simulink model "Automated_features"  (R2021a)
settings: Solver=VariableStepAuto  StartTime=0.0  StopTime=10.0  RelTol=1e-3
undefined symbols (not defined in the file): sigbuilder_block
libraries: simulink x123
(part 1 of 2)
settings Model: Creator=99003762  LastModifiedBy=Dell
settings SolverCC: AlgebraicLoopSolver=TrustRegion
settings DebuggingCC: SFMachineParentedDataDiag=warning

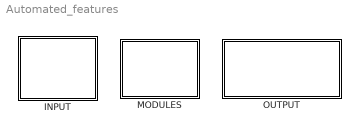
== system Automated_features ==
  INPUT : Subsystem
  MODULES : Subsystem
  OUTPUT : Subsystem

== system Automated_features/INPUT ==
  AIRBAG_INPUTS : Subsystem
  ALARM_INPUTS : Subsystem
  SEAT_RESTRAINT_INPUTS : Subsystem
  Wiper_INPUTS : Subsystem

== system Automated_features/MODULES ==
  AIRBAGSYSTEM : Subsystem
  ALARM_SYSTEM : Subsystem
  SeatBelt_MODULE : Subsystem
  WIPER_CONTROL : Subsystem
  tag scope: CushionAngle=global, FrontAngle=global, RearAngle=global, SeatAdj=global
  wires:
  SeatBelt_MODULE/4(CushionAdjustAngle) -> [CushionAngle]
  SeatBelt_MODULE/2(RearAdjustAngle) -> [RearAngle]
  SeatBelt_MODULE/3(SeatAdjust) -> [SeatAdj]
  SeatBelt_MODULE/1(FrontAdjustAngle) -> [FrontAngle]

== system Automated_features/OUTPUT ==
  AIRBAG_OUTPUTS : Subsystem
  ALARM_OUTPUT1 : Subsystem
  OUTPUT2 : Subsystem
  SeatBelt_OUTPUTS : Subsystem

== system Automated_features/INPUT/AIRBAG_INPUTS ==
  Signal Builder : Subsystem  Tag=STV Subsys  LoadFcn=sigbuilder_block('load');  StartFcn=sigbuilder_block('start');  StopFcn=sigbuilder_block('stop');  ClipboardFcn=sigbuilder_block('clipboard');  mask(Sigbuilder block){tuvar=[0:10]}
      mask help: Simulink:masks:SigbuilderBlock_MD
      mask init:
      | if ~strcmp(get_param(bdroot(gcbh),'SimulationStatus'),'stopped') tuvar = sigbuilder_block('maskInit'); end
      settings: CopyFcn=sigbuilder_block('copy');  DeleteFcn=sigbuilder_block('delete');  ModelCloseFcn=sigbuilder_block('modelClose');  PreSaveFcn=sigbuilder_block('preSave');  PauseFcn=sigbuilder_block('pause');  ContinueFcn=sigbuilder_block('continue');  NameChangeFcn=sigbuilder_block('namechange');  OpenFcn=sigbuilder_block('open',[437.6 199.2 550.4 400 ]);  CloseFcn=sigbuilder_block('close');
      mask Display: plot(0, 0, 100, 100,[2, 2, 32, 32, 2], [68, 8, 8, 68, 68],[32, 2], [38, 38], [32, 19, 2],[53, 60, 44], [32, 17, 17, 2],[16, 16, 31, 31]);txt = getActiveGroup(gcbh);text(2, 100, txt,'verticalAlignment', 'top');
  tag scope: Air_ACC=global, Driver_L=global, L_Front_1=global, L_Rear_1=global, R_Rear_=global, VehicleSpeed=global, YawRate=global
  wires:
  Signal Builder/1(Driver_L) -> [Driver_L]
  Signal Builder/2(L_Front_1) -> [L_Front_1]
  Signal Builder/3(L_Rear_1) -> [L_Rear_1]
  Signal Builder/4(R_Rear_) -> [R_Rear_]
  Signal Builder/5(VehicleSpeed) -> [VehicleSpeed]
  Signal Builder/6(Air_ACC) -> [Air_ACC]
  Signal Builder/7(YawRate) -> [YawRate]

== system Automated_features/INPUT/ALARM_INPUTS ==
  Signal Builder : Subsystem  Tag=STV Subsys  LoadFcn=sigbuilder_block('load');  StartFcn=sigbuilder_block('start');  StopFcn=sigbuilder_block('stop');  ClipboardFcn=sigbuilder_block('clipboard');  mask(Sigbuilder block){tuvar=[0:10]}
      mask help: Simulink:masks:SigbuilderBlock_MD
      mask init:
      | if ~strcmp(get_param(bdroot(gcbh),'SimulationStatus'),'stopped') tuvar = sigbuilder_block('maskInit'); end
      settings: CopyFcn=sigbuilder_block('copy');  DeleteFcn=sigbuilder_block('delete');  ModelCloseFcn=sigbuilder_block('modelClose');  PreSaveFcn=sigbuilder_block('preSave');  PauseFcn=sigbuilder_block('pause');  ContinueFcn=sigbuilder_block('continue');  NameChangeFcn=sigbuilder_block('namechange');  OpenFcn=sigbuilder_block('open',[403.5 199.2 550.5 359.55 ]);  CloseFcn=sigbuilder_block('close');
      mask Display: plot(0, 0, 100, 100,[2, 2, 32, 32, 2], [68, 8, 8, 68, 68],[32, 2], [38, 38], [32, 19, 2],[53, 60, 44], [32, 17, 17, 2],[16, 16, 31, 31]);txt = getActiveGroup(gcbh);text(2, 100, txt,'verticalAlignment', 'top');
  tag scope: AS_Doors=global, CAR_ON=global, Ignition=global, RKE=global
  wires:
  Signal Builder/1(AS_Doors) -> [AS_Doors]
  Signal Builder/2(Ignition) -> [Ignition]
  Signal Builder/3(Car_ON) -> [CAR_ON]
  Signal Builder/4(RKE) -> [RKE]

== system Automated_features/INPUT/SEAT_RESTRAINT_INPUTS ==
  tag scope: AdjustCushionAngle=global, AdjustFrontSeatAngle=global, AdjustRearSeatAngle=global, AdjustSeat=global, FrontSeat=global, HandleOn=global, ModeSelection=global, PowerSeat=global

== system Automated_features/INPUT/Wiper_INPUTS ==
  Signal Builder : Subsystem  Tag=STV Subsys  LoadFcn=sigbuilder_block('load');  StartFcn=sigbuilder_block('start');  StopFcn=sigbuilder_block('stop');  ClipboardFcn=sigbuilder_block('clipboard');  mask(Sigbuilder block){tuvar=[0:10]}
      mask help: Simulink:masks:SigbuilderBlock_MD
      mask init:
      | if ~strcmp(get_param(bdroot(gcbh),'SimulationStatus'),'stopped') tuvar = sigbuilder_block('maskInit'); end
      settings: CopyFcn=sigbuilder_block('copy');  DeleteFcn=sigbuilder_block('delete');  ModelCloseFcn=sigbuilder_block('modelClose');  PreSaveFcn=sigbuilder_block('preSave');  PauseFcn=sigbuilder_block('pause');  ContinueFcn=sigbuilder_block('continue');  NameChangeFcn=sigbuilder_block('namechange');  OpenFcn=sigbuilder_block('open',[437.6 199.2 550.4 400 ]);  CloseFcn=sigbuilder_block('close');
      mask Display: plot(0, 0, 100, 100,[2, 2, 32, 32, 2], [68, 8, 8, 68, 68],[32, 2], [38, 38], [32, 19, 2],[53, 60, 44], [32, 17, 17, 2],[16, 16, 31, 31]);txt = getActiveGroup(gcbh);text(2, 100, txt,'verticalAlignment', 'top');
  tag scope: FC_ManualInput=global, FW_Modes=global, WC_BackS=global, WC_FrontS=global, WC_Status=global
  wires:
  Signal Builder/1(FC_Modes) -> [FW_Modes]
  Signal Builder/2(FC_ManualInput) -> [FC_ManualInput]
  Signal Builder/3(WC_BackS) -> [WC_BackS]
  Signal Builder/4(WC_Fronts) -> [WC_FrontS]
  Signal Builder/5(WC_Status) -> [WC_Status]

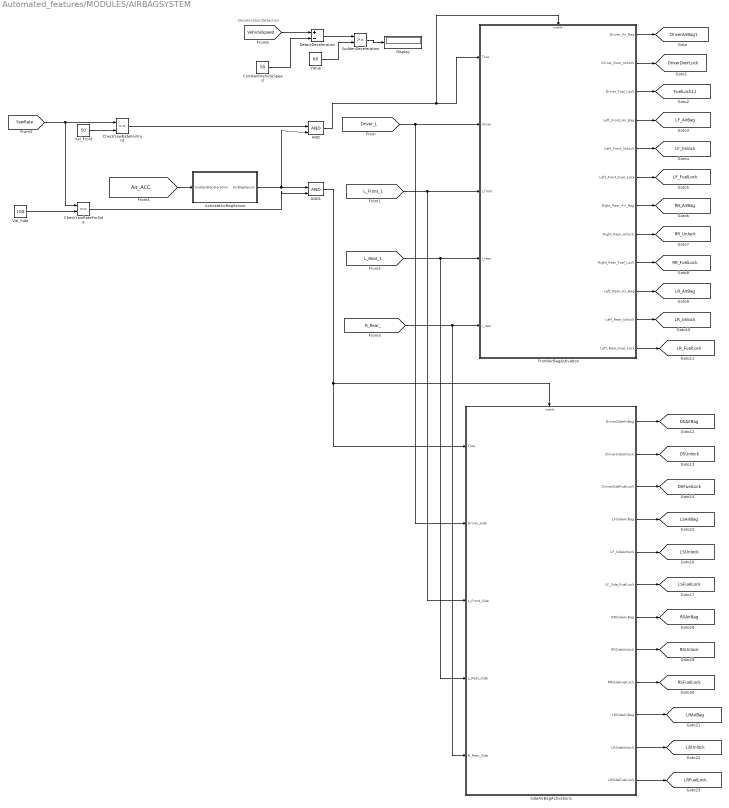
== system Automated_features/MODULES/AIRBAGSYSTEM ==
  note: DecelerationDetection
  AND : Logic  IconShape=distinctive  AllPortsSameDT=off  OutDataTypeStr=boolean
  AND1 : Logic  IconShape=distinctive  AllPortsSameDT=off  OutDataTypeStr=boolean
  ActivateAirBagSensor : MATLAB Function  TreatAsAtomicUnit=on
  CheckYawRateForFront : RelationalOperator  Operator===  OutDataTypeStr=boolean  RndMeth=Simplest
  CheckYawRateForSide : RelationalOperator  Operator===  OutDataTypeStr=boolean  RndMeth=Simplest
  ConstantVehicleSpeed : Constant  Value=50
  DetectDeceleration : Sum  Inputs=+-
  Display : Display
  FrontAirBagActivation : Subsystem  TreatAsAtomicUnit=on
  SideAirBagActivation1 : Subsystem  TreatAsAtomicUnit=on
  SuddenDeceleration : RelationalOperator  OutDataTypeStr=boolean  RndMeth=Simplest
  Val_Front : Constant  Value=50
  Val_Side : Constant  Value=100
  Value : Constant  Value=60
  tag scope: DSAirBag=global, DSFuelLock=global, DSUnlock=global, DriverAirBag1=global, DriverDoorLock=global, FuelLock11=global, LF_AirBag=global, LF_FuelLock=global, LF_Unlock=global, LRAirBag=global, LRFuelLock=global, LRUnlock=global, LR_AirBag=global, LR_FuelLock=global, LR_Unlock=global, LSAirBag=global, LSFuelLock=global, LSUnlock=global, RR_AirBag=global, RR_FuelLock=global, RR_Unlock=global, RSAirBag=global, RSFuelLock=global, RSUnlock=global
  wires:
  CheckYawRateForFront/1 -> AND/1
  AND1/1 -> SideAirBagActivation1/1(True), SideAirBagActivation1/Enable
  ActivateAirBagSensor/1(AirBagSensor) -> AND1/1, AND/2
  [VehicleSpeed] -> DetectDeceleration/1
  ConstantVehicleSpeed/1 -> DetectDeceleration/2
  AND/1 -> FrontAirBagActivation/1(True), FrontAirBagActivation/Enable
  [Air_ACC] -> ActivateAirBagSensor/1(SuddenDeceleration)
  Value/1 -> SuddenDeceleration/2
  DetectDeceleration/1 -> SuddenDeceleration/1
  SuddenDeceleration/1 -> Display/1
  [YawRate] -> CheckYawRateForSide/1, CheckYawRateForFront/1
  Val_Side/1 -> CheckYawRateForSide/2
  [Driver_L] -> FrontAirBagActivation/2(driver), SideAirBagActivation1/2(Driver_Side)
  Val_Front/1 -> CheckYawRateForFront/2
  [R_Rear_] -> SideAirBagActivation1/5(R_Rear_Side), FrontAirBagActivation/5(r_rear)
  [L_Rear_1] -> SideAirBagActivation1/4(L_Rear_Side), FrontAirBagActivation/4(l_rear)
  [L_Front_1] -> FrontAirBagActivation/3(l_front), SideAirBagActivation1/3(L_Front_Side)
  CheckYawRateForSide/1 -> AND1/2
  FrontAirBagActivation/1(Driver_Air_Bag) -> [DriverAirBag1]
  FrontAirBagActivation/2(Driver_Door_Unlock) -> [DriverDoorLock]
  FrontAirBagActivation/3(Driver_Fuel_Lock) -> [FuelLock11]
  FrontAirBagActivation/4(Left_Front_Air_Bag) -> [LF_AirBag]
  FrontAirBagActivation/5(Left_Front_Unlock) -> [LF_Unlock]
  FrontAirBagActivation/6(Left_Front_Fuel_Lock) -> [LF_FuelLock]
  FrontAirBagActivation/7(Right_Rear_Air_Bag) -> [RR_AirBag]
  FrontAirBagActivation/8(Right_Rear_Unlock) -> [RR_Unlock]
  FrontAirBagActivation/9(Right_Rear_Fuel_Lock) -> [RR_FuelLock]
  FrontAirBagActivation/10(Left_Rear_Air_Bag) -> [LR_AirBag]
  FrontAirBagActivation/11(Left_Rear_Unlock) -> [LR_Unlock]
  FrontAirBagActivation/12(Left_Rear_Fuel_Lock) -> [LR_FuelLock]
  SideAirBagActivation1/1(DriverSideAirBag) -> [DSAirBag]
  SideAirBagActivation1/2(DriverSideUnlock) -> [DSUnlock]
  SideAirBagActivation1/3(DriverSideFuelLock) -> [DSFuelLock]
  SideAirBagActivation1/4(LFSideAirBag) -> [LSAirBag]
  SideAirBagActivation1/5(LF_SideUnlock) -> [LSUnlock]
  SideAirBagActivation1/6(LF_Side_FuelLock) -> [LSFuelLock]
  SideAirBagActivation1/7(RRSideAirBag) -> [RSAirBag]
  SideAirBagActivation1/8(RRSideUnlock) -> [RSUnlock]
  SideAirBagActivation1/9(RRSideFuelLock) -> [RSFuelLock]
  SideAirBagActivation1/10(LRSideAirBag) -> [LRAirBag]
  SideAirBagActivation1/11(LRSideUnlock) -> [LRUnlock]
  SideAirBagActivation1/12(LRSideFuelLock) -> [LRFuelLock]

== system Automated_features/MODULES/ALARM_SYSTEM ==
  AND : Logic  Inputs=3  IconShape=distinctive  AllPortsSameDT=off  OutDataTypeStr=boolean
  AND1 : Logic  Inputs=3  IconShape=distinctive  AllPortsSameDT=off  OutDataTypeStr=boolean
  AND2 : Logic  IconShape=distinctive  AllPortsSameDT=off  OutDataTypeStr=boolean
  AND3 : Logic  IconShape=distinctive  AllPortsSameDT=off  OutDataTypeStr=boolean
  ARMED : Stateflow chart  TreatAsAtomicUnit=on
  Compare To Constant : simulink/Logic and Bit Operations/Compare To Constant  relop===  const=0  OutDataTypeStr=boolean
  Compare To Constant2 : simulink/Logic and Bit Operations/Compare To Constant  relop===  const=1  OutDataTypeStr=boolean
  Compare To Constant3 : simulink/Logic and Bit Operations/Compare To Constant  relop===  const=1  OutDataTypeStr=boolean
  Compare To Zero : simulink/Logic and Bit Operations/Compare To Zero  relop===  OutDataTypeStr=boolean
  Compare To Zero1 : simulink/Logic and Bit Operations/Compare To Zero  relop===  OutDataTypeStr=boolean
  Constant : Constant
  Constant1 : Constant
  Constant2 : Constant
  Constant3 : Constant  Value=0
  Display : Display
  Main_Alarm : Subsystem  Commented=on
  NAND : Logic  Operator=NAND  IconShape=distinctive  AllPortsSameDT=off  OutDataTypeStr=boolean
  Pre_Alarm : Stateflow chart  TreatAsAtomicUnit=on
  Slider Switch : SliderSwitchBlock  Commented=on
      settings: Values={{'Off', 'On'}, [1 0]}
  Switch : Switch  Criteria=u2 ~= 0
  Switch1 : Switch  Criteria=u2 ~= 0
  Switch2 : Switch  Criteria=u2 ~= 0
  tag scope: Alarm_ARMED=global, Disarmed=global, Prealarm_ARMED=global
  wires:
  [RKE] -> AND1/2, Compare To Zero/1, AND2/2  "RKE"
  Constant/1 -> Switch/1
  Constant1/1 -> Switch1/1
  Compare To Zero1/1 -> AND3/2
  Compare To Constant3/1 -> NAND/1
  [CAR_ON] -> AND/2
  Compare To Zero/1 -> AND3/1
  AND2/1 -> ARMED/1(data)
  Pre_Alarm/1(data1) -> Switch1/2
  Compare To Constant/1 -> AND2/1
  AND1/1 -> Switch/2
  [Ignition] -> Compare To Constant2/1, AND/1
  AND/1 -> Compare To Constant/1
  Compare To Constant2/1 -> AND1/1
  Switch/1 -> Switch2/2, [Disarmed]
  Switch1/1 -> [Prealarm_ARMED]
  ARMED/1(data1) -> AND1/3, Compare To Constant3/1
  AND3/1 -> Pre_Alarm/1(data)
  [AS_Doors] -> Display/1, Compare To Zero1/1, AND/3
  Constant2/1 -> Switch2/1
  Switch2/1 -> NAND/2
  NAND/1 -> [Alarm_ARMED]
  Constant3/1 -> Switch2/3

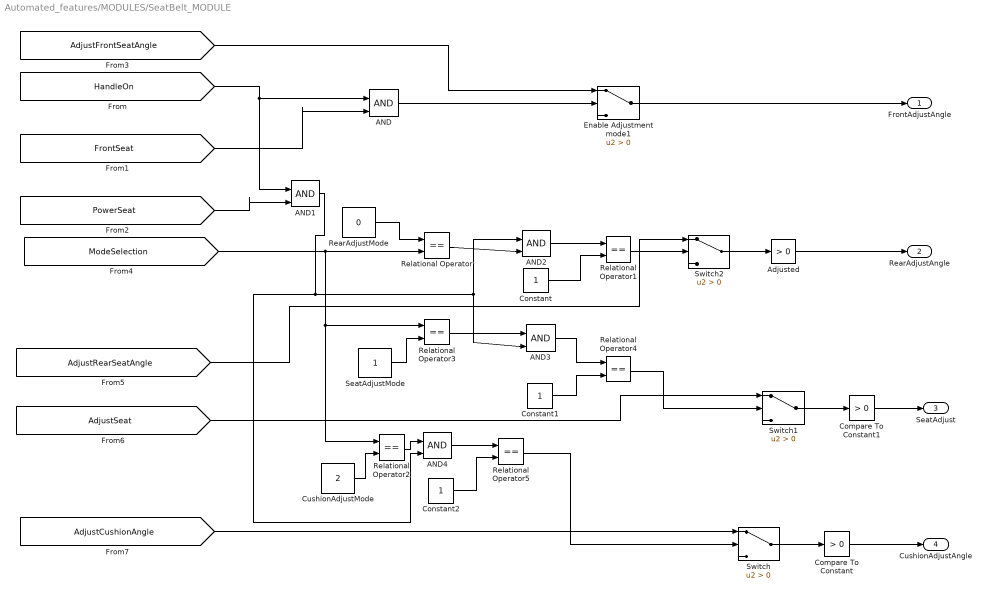
== system Automated_features/MODULES/SeatBelt_MODULE ==
  AND{,1..4} (5 alike) : Logic  IconShape=distinctive  AllPortsSameDT=off  OutDataTypeStr=boolean
  Adjusted : simulink/Logic and Bit Operations/Compare To Constant  relop=>  const=0  OutDataTypeStr=boolean
  Compare To Constant : simulink/Logic and Bit Operations/Compare To Constant  relop=>  const=0  OutDataTypeStr=boolean
  Compare To Constant1 : simulink/Logic and Bit Operations/Compare To Constant  relop=>  const=0  OutDataTypeStr=boolean
  Constant : Constant
  Constant1 : Constant
  Constant2 : Constant
  CushionAdjustMode : Constant  Value=2
  Enable Adjustment mode1 : Switch  Criteria=u2 > Threshold
  RearAdjustMode : Constant  Value=0
  Relational Operator{,1..5} (6 alike) : RelationalOperator  Operator===  OutDataTypeStr=boolean  RndMeth=Simplest
  SeatAdjustMode : Constant
  Switch : Switch  Criteria=u2 > Threshold
  Switch1 : Switch  Criteria=u2 > Threshold
  Switch2 : Switch  Criteria=u2 > Threshold
  FrontAdjustAngle : Outport
  RearAdjustAngle : Outport  Port=2
  SeatAdjust : Outport  Port=3
  CushionAdjustAngle : Outport  Port=4
  wires:
  AND3/1 -> Relational Operator4/1
  Compare To Constant/1 -> CushionAdjustAngle/1
  AND1/1 -> AND4/2, AND2/1, AND3/2
  [HandleOn] -> AND1/1, AND/1
  Switch2/1 -> Adjusted/1
  RearAdjustMode/1 -> Relational Operator/1
  [AdjustCushionAngle] -> Switch/1
  AND2/1 -> Relational Operator1/1
  AND/1 -> Enable Adjustment mode1/2
  Relational Operator2/1 -> AND4/1
  Compare To Constant1/1 -> SeatAdjust/1
  Constant/1 -> Relational Operator1/2
  [AdjustSeat] -> Switch1/1
  Relational Operator4/1 -> Switch1/2
  Switch/1 -> Compare To Constant/1
  Switch1/1 -> Compare To Constant1/1
  Relational Operator/1 -> AND2/2
  [FrontSeat] -> AND/2
  [AdjustRearSeatAngle] -> Switch2/1
  [ModeSelection] -> Relational Operator/2, Relational Operator2/1, Relational Operator3/1
  AND4/1 -> Relational Operator5/1
  Relational Operator3/1 -> AND3/1
  SeatAdjustMode/1 -> Relational Operator3/2
  Constant2/1 -> Relational Operator5/2
  Constant1/1 -> Relational Operator4/2
  [AdjustFrontSeatAngle] -> Enable Adjustment mode1/1
  Relational Operator1/1 -> Switch2/2
  Relational Operator5/1 -> Switch/2
  CushionAdjustMode/1 -> Relational Operator2/2
  [PowerSeat] -> AND1/2
  Adjusted/1 -> RearAdjustAngle/1
  Enable Adjustment mode1/1 -> FrontAdjustAngle/1

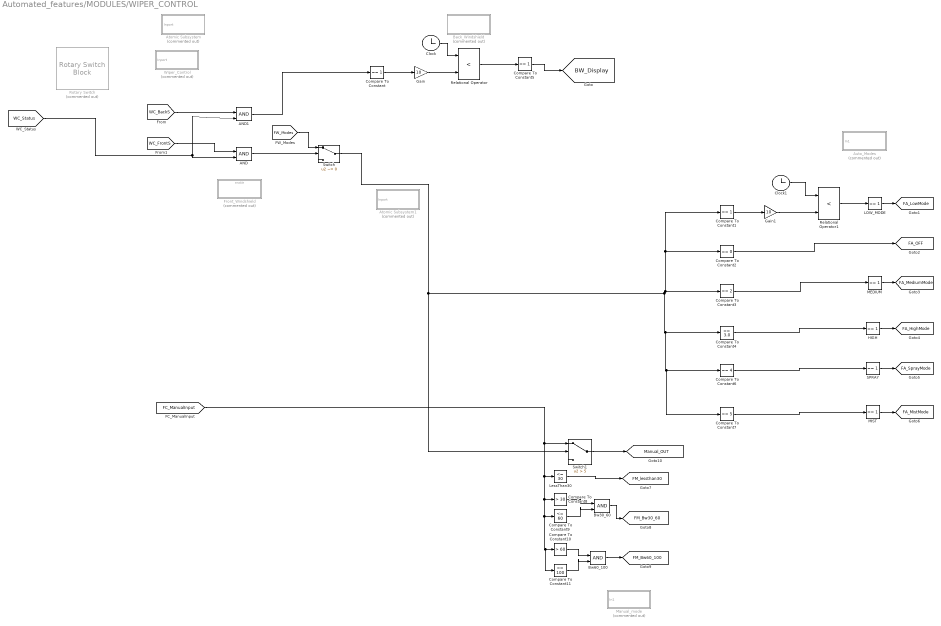
== system Automated_features/MODULES/WIPER_CONTROL ==
  AND : Logic  IconShape=distinctive  AllPortsSameDT=off  OutDataTypeStr=boolean
  AND1 : Logic  IconShape=distinctive  AllPortsSameDT=off  OutDataTypeStr=boolean
  Atomic Subsystem : Subsystem  Commented=on  TreatAsAtomicUnit=on
  Atomic Subsystem1 : Subsystem  Commented=on  TreatAsAtomicUnit=on
  Auto_Modes : Subsystem  Commented=on
  Back_Windshield : Subsystem  Commented=on  TreatAsAtomicUnit=on
  Bw30_60 : Logic  IconShape=distinctive  AllPortsSameDT=off  OutDataTypeStr=boolean
  Bw60_100 : Logic  IconShape=distinctive  AllPortsSameDT=off  OutDataTypeStr=boolean
  Clock : Clock
      settings: Decimation=5
  Clock1 : Clock
      settings: Decimation=5
  Compare To Constant : simulink/Logic and Bit Operations/Compare To Constant  relop===  const=1  OutDataTypeStr=boolean
  Compare To Constant1 : simulink/Logic and Bit Operations/Compare To Constant  relop===  const=1  OutDataTypeStr=boolean
  Compare To Constant10 : simulink/Logic and Bit Operations/Compare To Constant  relop=>  const=60  OutDataTypeStr=boolean
  Compare To Constant11 : simulink/Logic and Bit Operations/Compare To Constant  relop=<=  const=100  OutDataTypeStr=boolean
  Compare To Constant2 : simulink/Logic and Bit Operations/Compare To Constant  relop===  const=0  OutDataTypeStr=boolean
  Compare To Constant3 : simulink/Logic and Bit Operations/Compare To Constant  relop===  const=2  OutDataTypeStr=boolean
  Compare To Constant4 : simulink/Logic and Bit Operations/Compare To Constant  relop===  const=3.0  OutDataTypeStr=boolean
  Compare To Constant5 : simulink/Logic and Bit Operations/Compare To Constant  relop===  const=1  OutDataTypeStr=boolean
  Compare To Constant6 : simulink/Logic and Bit Operations/Compare To Constant  relop===  const=4  OutDataTypeStr=boolean
  Compare To Constant7 : simulink/Logic and Bit Operations/Compare To Constant  relop===  const=5  OutDataTypeStr=boolean
  Compare To Constant8 : simulink/Logic and Bit Operations/Compare To Constant  relop=>  const=30  OutDataTypeStr=boolean
  Compare To Constant9 : simulink/Logic and Bit Operations/Compare To Constant  relop=<=  const=60  OutDataTypeStr=boolean
  Front_Windshield : Subsystem  Commented=on  TreatAsAtomicUnit=on
  Gain : Gain  Gain=10
  Gain1 : Gain  Gain=10
  HIGH : simulink/Logic and Bit Operations/Compare To Constant  relop===  const=1  OutDataTypeStr=boolean
  LOW_MODE : simulink/Logic and Bit Operations/Compare To Constant  relop===  const=1  OutDataTypeStr=boolean
  LessThan30 : simulink/Logic and Bit Operations/Compare To Constant  relop=<=  const=30  OutDataTypeStr=boolean
  MEDIUM : simulink/Logic and Bit Operations/Compare To Constant  relop===  const=1  OutDataTypeStr=boolean
  MIST : simulink/Logic and Bit Operations/Compare To Constant  relop===  const=1  OutDataTypeStr=boolean
  Manual_mode : Subsystem  Commented=on
  Relational Operator : RelationalOperator  Operator=<  OutDataTypeStr=boolean  RndMeth=Simplest
  Relational Operator1 : RelationalOperator  Operator=<  OutDataTypeStr=boolean  RndMeth=Simplest
  Rotary Switch : RotarySwitchBlock  Commented=on
      settings: Values={{'Off', 'Accessory', 'Ignition'}, [0 1 2]}
  SPRAY : simulink/Logic and Bit Operations/Compare To Constant  relop===  const=1  OutDataTypeStr=boolean
  Switch : Switch  Criteria=u2 ~= 0
  Switch1 : Switch  Criteria=u2 > Threshold  Threshold=5
  Wiper_Control : Subsystem  Commented=on  TreatAsAtomicUnit=on
  tag scope: BW_Display=global, FA_HighMode=global, FA_LowMode=global, FA_MediumMode=global, FA_MistMode=global, FA_OFF=global, FA_SprayMode=global, FM_Bw30_60=global, FM_Bw60_100=global, FM_lessthan30=global, Manual_OUT=global
  wires:
  [WC_Status] -> AND1/2, AND/2
  [WC_BackS] -> AND1/1
  [WC_FrontS] -> AND/1
  Compare To Constant/1 -> Gain/1
  Relational Operator/1 -> Compare To Constant5/1
  Compare To Constant5/1 -> [BW_Display]
  Gain/1 -> Relational Operator/2
  Clock/1 -> Relational Operator/1
  AND1/1 -> Compare To Constant/1
  AND/1 -> Switch/2
  [FW_Modes] -> Switch/1
  Compare To Constant6/1 -> SPRAY/1
  MEDIUM/1 -> [FA_MediumMode]
  HIGH/1 -> [FA_HighMode]
  LOW_MODE/1 -> [FA_LowMode]
  Relational Operator1/1 -> LOW_MODE/1
  Clock1/1 -> Relational Operator1/1
  Gain1/1 -> Relational Operator1/2
  SPRAY/1 -> [FA_SprayMode]
  MIST/1 -> [FA_MistMode]
  Compare To Constant7/1 -> MIST/1
  Compare To Constant2/1 -> [FA_OFF]
  Compare To Constant1/1 -> Gain1/1
  Switch1/1 -> [Manual_OUT]
  [FC_ManualInput] -> Compare To Constant11/1, Compare To Constant10/1, Compare To Constant9/1, Compare To Constant8/1, LessThan30/1, Switch1/1
  Compare To Constant9/1 -> Bw30_60/2
  Switch/1 -> Switch1/2, Compare To Constant7/1, Compare To Constant6/1, Compare To Constant4/1, Compare To Constant3/1, Compare To Constant1/1, Compare To Constant2/1
  LessThan30/1 -> [FM_lessthan30]
  Compare To Constant10/1 -> Bw60_100/1
  Compare To Constant8/1 -> Bw30_60/1
  Compare To Constant11/1 -> Bw60_100/2
  Bw60_100/1 -> [FM_Bw60_100]
  Bw30_60/1 -> [FM_Bw30_60]
  Compare To Constant3/1 -> MEDIUM/1
  Compare To Constant4/1 -> HIGH/1

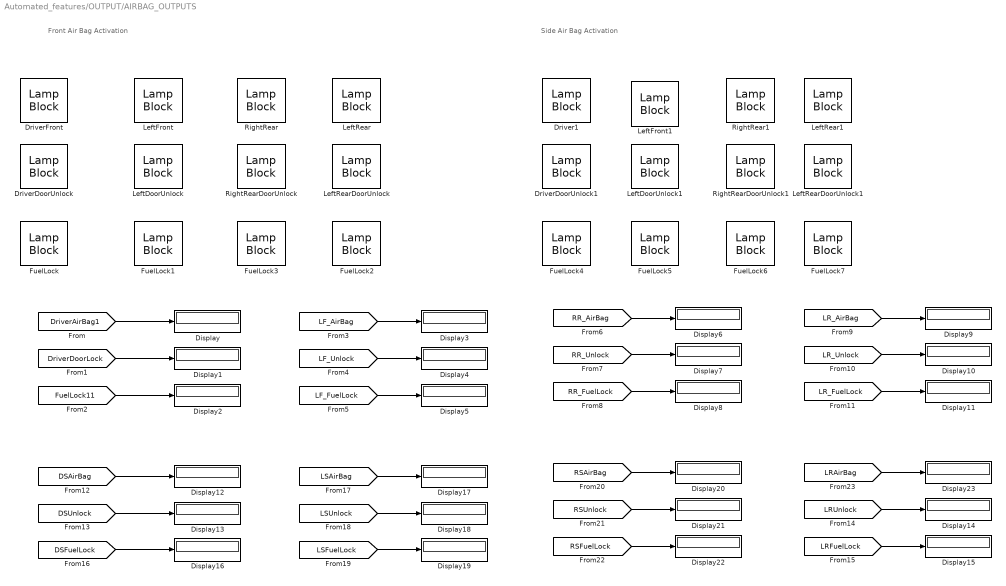
== system Automated_features/OUTPUT/AIRBAG_OUTPUTS ==
  note: Front Air Bag Activation
  note: Side Air Bag Activation
  Display{,1..23} (24 alike) : Display
  Driver1 : LampBlock
  DriverDoorUnlock : LampBlock
  DriverDoorUnlock1 : LampBlock
  DriverFront : LampBlock  Icon=Circle
  FuelLock{,1..7} (8 alike) : LampBlock
  LeftDoorUnlock : LampBlock
  LeftDoorUnlock1 : LampBlock
  LeftFront : LampBlock
  LeftFront1 : LampBlock
  LeftRear : LampBlock
  LeftRear1 : LampBlock
  LeftRearDoorUnlock : LampBlock
  LeftRearDoorUnlock1 : LampBlock
  RightRear : LampBlock
  RightRear1 : LampBlock
  RightRearDoorUnlock : LampBlock
  RightRearDoorUnlock1 : LampBlock
  wires:
  [DriverAirBag1] -> Display/1
  [DriverDoorLock] -> Display1/1
  [FuelLock11] -> Display2/1
  [LF_AirBag] -> Display3/1
  [LF_Unlock] -> Display4/1
  [LF_FuelLock] -> Display5/1
  [RR_AirBag] -> Display6/1
  [RR_Unlock] -> Display7/1
  [RR_FuelLock] -> Display8/1
  [LR_AirBag] -> Display9/1
  [LR_Unlock] -> Display10/1
  [LR_FuelLock] -> Display11/1
  [DSFuelLock] -> Display16/1
  [LRAirBag] -> Display23/1
  [RSUnlock] -> Display21/1
  [RSAirBag] -> Display20/1
  [RSFuelLock] -> Display22/1
  [DSUnlock] -> Display13/1
  [LSUnlock] -> Display18/1
  [LRUnlock] -> Display14/1
  [LSFuelLock] -> Display19/1
  [LSAirBag] -> Display17/1
  [LRFuelLock] -> Display15/1
  [DSAirBag] -> Display12/1

== system Automated_features/OUTPUT/ALARM_OUTPUT1 ==
  note: OUTPUTS
  Display : Display
  Display1 : Display
  Display2 : Display
  Lamp : LampBlock
  wires:
  [Disarmed] -> Display2/1
  [Prealarm_ARMED] -> Display1/1
  [Alarm_ARMED] -> Display/1

== system Automated_features/OUTPUT/OUTPUT2 ==
  note: BACK WINDSHIELD
  note: FRONT WINDSHIELD AUTOMODES
  note: FRONT WINDSHIELD MANUAL MANUAL OUTPUT
  Display{,1..10} (11 alike) : Display
  Lamp{,1..8} (9 alike) : LampBlock
  wires:
  [BW_Display] -> Display/1
  [FM_lessthan30] -> Display1/1
  [FM_Bw30_60] -> Display2/1
  [FM_Bw60_100] -> Display3/1
  [FA_LowMode] -> Display4/1
  [FA_MediumMode] -> Display5/1
  [FA_HighMode] -> Display6/1
  [FA_MistMode] -> Display7/1
  [FA_OFF] -> Display8/1
  [FA_SprayMode] -> Display9/1
  [Manual_OUT] -> Display10/1

== system Automated_features/OUTPUT/SeatBelt_OUTPUTS ==
  Display{,1..3} (4 alike) : Display
  wires:
  [RearAngle] -> Display1/1
  [SeatAdj] -> Display2/1
  [FrontAngle] -> Display/1
  [CushionAngle] -> Display3/1

== system Automated_features/INPUT/AIRBAG_INPUTS/Signal Builder ==
  Demux : Demux  Tag=STV Demux  Outputs=7
      settings: DisplayOption=none
  FromWs : FromWorkspace  Tag=STV FromWs  VariableName=tuvar
      SigBuilderData=|
      | common.afterFinalStr = 'Extrapolate'
      | common.sampleTime = 0
      | dataSet.timeRange = [0 10]
      | dataSet.name = 'Group 1'
      | sbobj.Groups.Name = 'Group 1'
      | sbobj.Groups.Signals(1).Name = 'Driver_L'
      | sbobj.Groups.Signals(1).XData = [0 1 2 3 4 5 6 7 10]
      | sbobj.Groups.Signals(1).YData = [0 1 1 1 1 1 1 0 0]
      | sbobj.Groups.Signals(2).Name = 'L_Front_1'
      | sbobj.Groups.Signals(2).XData = [0 1 2 3 4 5 6 7 10]
      | sbobj.Groups.Signals(2).YData = [0 0 0 0 0 0 0 0 0]
      | sbobj.Groups.Signals(3).Name = 'L_Rear_1'
      | sbobj.Groups.Signals(3).XData = [0 1 2 3 4 5 6 7 10]
      | sbobj.Groups.Signals(3).YData = [0 0 0 0 0 0 0 0 0]
      | sbobj.Groups.Signals(4).Name = 'R_Rear_'
      | sbobj.Groups.Signals(4).XData = [0 1 2 3 4 5 6 7 10]
      | sbobj.Groups.Signals(4).YData = [0 0 0 0 0 0 0 1 1]
      | sbobj.Groups.Signals(5).Name = 'VehicleSpeed'
      | sbobj.Groups.Signals(5).XData = [0 1 2 3 4 5 6 7 10]
      | sbobj.Groups.Signals(5).YData = [0 50 50 140 140 140 140 140 140]
      | sbobj.Groups.Signals(6).Name = 'Air_ACC'
      | sbobj.Groups.Signals(6).XData = [0 1 2 3 4 5 6 7 10]
      | sbobj.Groups.Signals(6).YData = [0 0 0 1 1 1 1 1 1]
      | sbobj.Groups.Signals(7).Name = 'YawRate'
      | sbobj.Groups.Signals(7).XData = [0 1 2 3 4 5 6 7 8 10]
      | sbobj.Groups.Signals(7).YData = [0 50 50 50 50 100 100 50 100 100]
  Driver_L : Outport  Tag=STV Outport
  L_Front_1 : Outport  Tag=STV Outport  Port=2
  L_Rear_1 : Outport  Tag=STV Outport  Port=3
  R_Rear_ : Outport  Tag=STV Outport  Port=4
  VehicleSpeed : Outport  Tag=STV Outport  Port=5
  Air_ACC : Outport  Tag=STV Outport  Port=6
  YawRate : Outport  Tag=STV Outport  Port=7
  wires:
  FromWs/1 -> Demux/1
  Demux/1 -> Driver_L/1
  Demux/2 -> L_Front_1/1
  Demux/3 -> L_Rear_1/1
  Demux/4 -> R_Rear_/1
  Demux/5 -> VehicleSpeed/1
  Demux/6 -> Air_ACC/1
  Demux/7 -> YawRate/1

== system Automated_features/INPUT/ALARM_INPUTS/Signal Builder ==
  Demux : Demux  Tag=STV Demux
      settings: DisplayOption=none
  FromWs : FromWorkspace  Tag=STV FromWs  VariableName=tuvar
      SigBuilderData=|
      | common.afterFinalStr = 'Extrapolate'
      | common.sampleTime = 0
      | dataSet.timeRange = [0 12]
      | dataSet.name = 'Group 1'
      | sbobj.Groups.Name = 'Group 1'
      | sbobj.Groups.Signals(1).Name = 'AS_Doors'
      | sbobj.Groups.Signals(1).XData = [0 1 2 3 4 5 6 7 8 9 10 11 12]
      | sbobj.Groups.Signals(1).YData = [0 1 1 1 1 1 1 1 1 1 1 1 1]
      | sbobj.Groups.Signals(2).Name = 'Ignition'
      | sbobj.Groups.Signals(2).XData = [0 1 2 3 4 5 6 7 8 9 10 11 12]
      | sbobj.Groups.Signals(2).YData = [0 1 1 1 1 1 1 1 1 1 1 1 1]
      | sbobj.Groups.Signals(3).Name = 'Car_ON'
      | sbobj.Groups.Signals(3).XData = [0 1 2 3 4 5 6 7 8 9 10 11 12]
      | sbobj.Groups.Signals(3).YData = [0 1 1 1 1 1 1 1 1 1 1 1 1]
      | sbobj.Groups.Signals(4).Name = 'RKE'
      | sbobj.Groups.Signals(4).XData = [0 1 2 3 4 5 6 7 8 9 10 11 12]
      | sbobj.Groups.Signals(4).YData = [0 1 1 1 1 1 2 2 2 2 2 2 2]
      | sbobj.Groups.TimeRange = [0 12]
  AS_Doors : Outport  Tag=STV Outport
  Ignition : Outport  Tag=STV Outport  Port=2
  Car_ON : Outport  Tag=STV Outport  Port=3
  RKE : Outport  Tag=STV Outport  Port=4
  wires:
  FromWs/1 -> Demux/1
  Demux/1 -> AS_Doors/1
  Demux/2 -> Ignition/1
  Demux/3 -> Car_ON/1
  Demux/4 -> RKE/1

== system Automated_features/INPUT/Wiper_INPUTS/Signal Builder ==
  Demux : Demux  Tag=STV Demux  Outputs=5
      settings: DisplayOption=none
  FromWs : FromWorkspace  Tag=STV FromWs  VariableName=tuvar
      SigBuilderData=|
      | common.afterFinalStr = 'Extrapolate'
      | common.sampleTime = 0
      | dataSet.timeRange = [0 10]
      | dataSet.name = 'Group 1'
      | sbobj.Groups.Name = 'Group 1'
      | sbobj.Groups.Signals(1).Name = 'FC_Modes'
      | sbobj.Groups.Signals(1).XData = [0 1 2 3 4 5 6 7 8 9 10 11 12 13 14 15 16 17 18 19 20 21 22 23 24 25 26 27 28 29 30 31 32 33 34 35 36 37 38 39 40 41 42 43]
      | sbobj.Groups.Signals(1).YData = [0 1 1 1 1 1 1 1 1 1 1 1 2 2 2 2 2 2 2 2 3 3 3 3 3 4 4 4 4 4 5 5 5 6 6 6 6 6 6 6 6 6 6 6]
      | sbobj.Groups.Signals(2).Name = 'FC_ManualInput'
      | sbobj.Groups.Signals(2).XData = [0 1 2 3 4 5 6 7 8 9 10 11 12 13 14 15 16 17 18 19 20 21 22 23 24 25 26 27 28 29 30 31 32 33 34 35 36 37 38 39 40 41 42 43]
      | sbobj.Groups.Signals(2).YData = [0 0 0 0 0 0 0 0 0 0 0 0 0 0 0 0 0 0 0 0 0 0 0 0 0 0 0 0 0 0 0 0 0 0 15 20 36 50 65 69 80 85 90 98]
      | sbobj.Groups.Signals(3).Name = 'WC_BackS'
      | sbobj.Groups.Signals(3).XData = [0 1 2 3 4 5 6 7 8 9 10 11 12 13 14 15 16 17 18 19 20 21 22 23 24 25 26 27 28 29 30 31 32 33 34 35 36 37 38 39 40 41 42 43]
      | sbobj.Groups.Signals(3).YData = [0 1 1 1 1 1 1 1 1 1 1 1 0 0 0 0 0 0 0 0 0 0 0 0 0 0 0 0 0 0 0 0 0 0 0 0 0 0 0 0 0 0 0 0]
      | sbobj.Groups.Signals(4).Name = 'WC_Fronts'
      | sbobj.Groups.Signals(4).XData = [0 1 2 3 4 5 6 7 8 9 10 11 12 13 14 15 16 17 18 19 20 21 22 23 24 25 26 27 28 29 30 31 32 33 34 35 36 37 38 39 40 41 42 43]
      | sbobj.Groups.Signals(4).YData = [0 1 1 1 1 1 1 1 1 1 1 1 1 1 1 1 1 1 1 1 1 1 1 1 1 1 1 1 1 1 1 1 1 1 1 1 1 1 1 1 1 1 1 1]
      | sbobj.Groups.Signals(5).Name = 'WC_Status'
      | sbobj.Groups.Signals(5).XData = [0 1 2 3 4 5 6 7 8 9 10 11 12 13 14 15 16 17 18 19 20 21 22 23 24 25 26 27 28 29 30 31 32 33 34 35 36 37 38 39 40 41 42 43]
      | sbobj.Groups.Signals(5).YData = [0 1 1 1 1 1 1 1 1 1 1 1 1 1 1 1 1 1 1 1 1 1 1 1 1 1 1 1 1 1 1 1 1 1 1 1 1 1 1 1 1 1 1 1]
  FC_Modes : Outport  Tag=STV Outport
  FC_ManualInput : Outport  Tag=STV Outport  Port=2
  WC_BackS : Outport  Tag=STV Outport  Port=3
  WC_Fronts : Outport  Tag=STV Outport  Port=4
  WC_Status : Outport  Tag=STV Outport  Port=5
  wires:
  FromWs/1 -> Demux/1
  Demux/1 -> FC_Modes/1
  Demux/2 -> FC_ManualInput/1
  Demux/3 -> WC_BackS/1
  Demux/4 -> WC_Fronts/1
  Demux/5 -> WC_Status/1

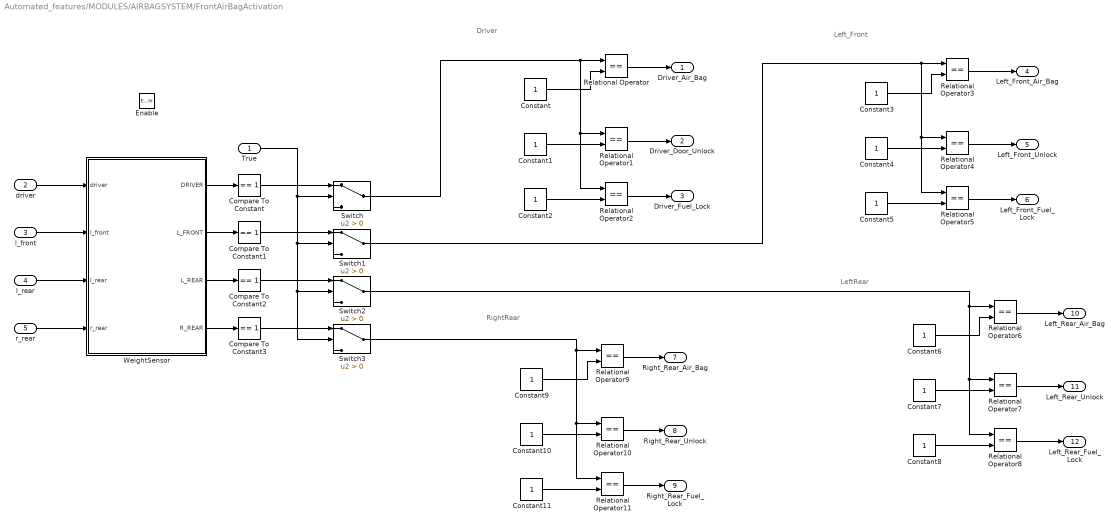
== system Automated_features/MODULES/AIRBAGSYSTEM/FrontAirBagActivation ==
  note: RightRear
  note: LeftRear
  note: Left_Front
  note: Driver
  True : Inport
  driver : Inport  Port=2
  l_front : Inport  Port=3
  l_rear : Inport  Port=4
  r_rear : Inport  Port=5
  Enable : EnablePort
  Compare To Constant{,1..3} (4 alike) : simulink/Logic and Bit Operations/Compare To Constant  relop===  const=1  OutDataTypeStr=boolean
  Constant{,1..11} (12 alike) : Constant
  Relational Operator{,1..11} (12 alike) : RelationalOperator  Operator===  OutDataTypeStr=boolean  RndMeth=Simplest
  Switch{,1..3} (4 alike) : Switch  Criteria=u2 > Threshold
  WeightSensor : MATLAB Function  TreatAsAtomicUnit=on
  Driver_Air_Bag : Outport
  Driver_Door_Unlock : Outport  Port=2
  Driver_Fuel_Lock : Outport  Port=3
  Left_Front_Air_Bag : Outport  Port=4
  Left_Front_Unlock : Outport  Port=5
  Left_Front_Fuel_Lock : Outport  Port=6
  Right_Rear_Air_Bag : Outport  Port=7
  Right_Rear_Unlock : Outport  Port=8
  Right_Rear_Fuel_Lock : Outport  Port=9
  Left_Rear_Air_Bag : Outport  Port=10
  Left_Rear_Unlock : Outport  Port=11
  Left_Rear_Fuel_Lock : Outport  Port=12
  wires:
  WeightSensor/2(L_FRONT) -> Compare To Constant1/1
  WeightSensor/1(DRIVER) -> Compare To Constant/1
  WeightSensor/3(L_REAR) -> Compare To Constant2/1
  WeightSensor/4(R_REAR) -> Compare To Constant3/1
  True/1 -> Switch3/2, Switch2/2, Switch1/2, Switch/2
  Compare To Constant/1 -> Switch/1
  Compare To Constant1/1 -> Switch1/1
  Compare To Constant2/1 -> Switch2/1
  Compare To Constant3/1 -> Switch3/1
  Constant2/1 -> Relational Operator2/2
  Switch/1 -> Relational Operator2/1, Relational Operator1/1, Relational Operator/1
  Constant1/1 -> Relational Operator1/2
  Constant/1 -> Relational Operator/2
  Constant4/1 -> Relational Operator4/2
  Constant5/1 -> Relational Operator5/2
  Switch1/1 -> Relational Operator5/1, Relational Operator4/1, Relational Operator3/1
  Constant3/1 -> Relational Operator3/2
  Constant7/1 -> Relational Operator7/2
  Constant6/1 -> Relational Operator6/2
  Switch2/1 -> Relational Operator8/1, Relational Operator7/1, Relational Operator6/1
  Constant8/1 -> Relational Operator8/2
  Switch3/1 -> Relational Operator11/1, Relational Operator10/1, Relational Operator9/1
  Constant11/1 -> Relational Operator11/2
  Constant10/1 -> Relational Operator10/2
  Constant9/1 -> Relational Operator9/2
  driver/1 -> WeightSensor/1(driver)
  l_front/1 -> WeightSensor/2(l_front)
  l_rear/1 -> WeightSensor/3(l_rear)
  r_rear/1 -> WeightSensor/4(r_rear)
  Relational Operator3/1 -> Left_Front_Air_Bag/1
  Relational Operator4/1 -> Left_Front_Unlock/1
  Relational Operator5/1 -> Left_Front_Fuel_Lock/1
  Relational Operator9/1 -> Right_Rear_Air_Bag/1
  Relational Operator10/1 -> Right_Rear_Unlock/1
  Relational Operator11/1 -> Right_Rear_Fuel_Lock/1
  Relational Operator6/1 -> Left_Rear_Air_Bag/1
  Relational Operator7/1 -> Left_Rear_Unlock/1
  Relational Operator8/1 -> Left_Rear_Fuel_Lock/1
  Relational Operator/1 -> Driver_Air_Bag/1
  Relational Operator1/1 -> Driver_Door_Unlock/1
  Relational Operator2/1 -> Driver_Fuel_Lock/1

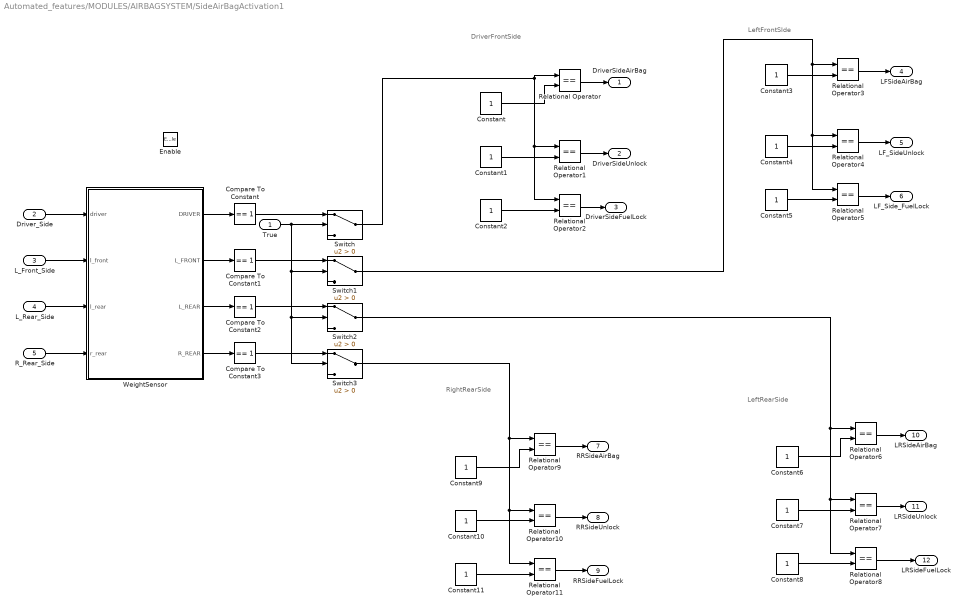
== system Automated_features/MODULES/AIRBAGSYSTEM/SideAirBagActivation1 ==
  note: RightRearSide
  note: LeftRearSide
  note: LeftFrontSIde
  note: DriverFrontSide
  True : Inport
  Driver_Side : Inport  Port=2
  L_Front_Side : Inport  Port=3
  L_Rear_Side : Inport  Port=4
  R_Rear_Side : Inport  Port=5
  Enable : EnablePort
  Compare To Constant{,1..3} (4 alike) : simulink/Logic and Bit Operations/Compare To Constant  relop===  const=1  OutDataTypeStr=boolean
  Constant{,1..11} (12 alike) : Constant
  Relational Operator{,1..11} (12 alike) : RelationalOperator  Operator===  OutDataTypeStr=boolean  RndMeth=Simplest
  Switch{,1..3} (4 alike) : Switch  Criteria=u2 > Threshold
  WeightSensor : MATLAB Function  TreatAsAtomicUnit=on
  DriverSideAirBag : Outport
  DriverSideUnlock : Outport  Port=2
  DriverSideFuelLock : Outport  Port=3
  LFSideAirBag : Outport  Port=4
  LF_SideUnlock : Outport  Port=5
  LF_Side_FuelLock : Outport  Port=6
  RRSideAirBag : Outport  Port=7
  RRSideUnlock : Outport  Port=8
  RRSideFuelLock : Outport  Port=9
  LRSideAirBag : Outport  Port=10
  LRSideUnlock : Outport  Port=11
  LRSideFuelLock : Outport  Port=12
  wires:
  WeightSensor/2(L_FRONT) -> Compare To Constant1/1
  WeightSensor/3(L_REAR) -> Compare To Constant2/1
  WeightSensor/4(R_REAR) -> Compare To Constant3/1
  Compare To Constant1/1 -> Switch1/1
  True/1 -> Switch3/2, Switch2/2, Switch1/2, Switch/2
  WeightSensor/1(DRIVER) -> Compare To Constant/1
  Compare To Constant3/1 -> Switch3/1
  Compare To Constant2/1 -> Switch2/1
  Compare To Constant/1 -> Switch/1
  Driver_Side/1 -> WeightSensor/1(driver)
  R_Rear_Side/1 -> WeightSensor/4(r_rear)
  L_Rear_Side/1 -> WeightSensor/3(l_rear)
  L_Front_Side/1 -> WeightSensor/2(l_front)
  Constant2/1 -> Relational Operator2/2
  Constant1/1 -> Relational Operator1/2
  Constant/1 -> Relational Operator/2
  Switch/1 -> Relational Operator2/1, Relational Operator1/1, Relational Operator/1
  Constant4/1 -> Relational Operator4/2
  Constant3/1 -> Relational Operator3/2
  Constant5/1 -> Relational Operator5/2
  Switch1/1 -> Relational Operator5/1, Relational Operator4/1, Relational Operator3/1
  Constant8/1 -> Relational Operator8/2
  Switch2/1 -> Relational Operator8/1, Relational Operator7/1, Relational Operator6/1
  Constant7/1 -> Relational Operator7/2
  Constant6/1 -> Relational Operator6/2
  Constant11/1 -> Relational Operator11/2
  Switch3/1 -> Relational Operator11/1, Relational Operator10/1, Relational Operator9/1
  Constant9/1 -> Relational Operator9/2
  Constant10/1 -> Relational Operator10/2
  Relational Operator/1 -> DriverSideAirBag/1
  Relational Operator1/1 -> DriverSideUnlock/1
  Relational Operator2/1 -> DriverSideFuelLock/1
  Relational Operator3/1 -> LFSideAirBag/1
  Relational Operator4/1 -> LF_SideUnlock/1
  Relational Operator5/1 -> LF_Side_FuelLock/1
  Relational Operator9/1 -> RRSideAirBag/1
  Relational Operator10/1 -> RRSideUnlock/1
  Relational Operator11/1 -> RRSideFuelLock/1
  Relational Operator6/1 -> LRSideAirBag/1
  Relational Operator7/1 -> LRSideUnlock/1
  Relational Operator8/1 -> LRSideFuelLock/1

== system Automated_features/MODULES/ALARM_SYSTEM/Main_Alarm ==
  data2 : Inport
  AND : Logic  Inputs=3  IconShape=distinctive  AllPortsSameDT=off  OutDataTypeStr=boolean
  AND1 : Logic  Inputs=3  IconShape=distinctive  AllPortsSameDT=off  OutDataTypeStr=boolean
  AND2 : Logic  IconShape=distinctive  AllPortsSameDT=off  OutDataTypeStr=boolean
  AND3 : Logic  IconShape=distinctive  AllPortsSameDT=off  OutDataTypeStr=boolean
  ARMED : Stateflow chart  TreatAsAtomicUnit=on
  Compare To Constant : simulink/Logic and Bit Operations/Compare To Constant  relop===  const=0  OutDataTypeStr=boolean
  Compare To Constant2 : simulink/Logic and Bit Operations/Compare To Constant  relop===  const=1  OutDataTypeStr=boolean
  Compare To Constant3 : simulink/Logic and Bit Operations/Compare To Constant  relop===  const=1  OutDataTypeStr=boolean
  Compare To Zero : simulink/Logic and Bit Operations/Compare To Zero  relop===  OutDataTypeStr=boolean
  Compare To Zero1 : simulink/Logic and Bit Operations/Compare To Zero  relop===  OutDataTypeStr=boolean
  Display3 : DisplayBlock  LabelPosition=Hide  Format=short  Transparency=1
  Display4 : DisplayBlock  LabelPosition=Hide  Format=short  Transparency=1
  Lamp : LampBlock
  Pre_Alarm : Stateflow chart  TreatAsAtomicUnit=on
  Rotary Switch : RotarySwitchBlock
      settings: Values={{'zero', 'one', 'Unlocking'}, [0 1 2]}
  String Constant : StringConstant  String="\"DISARMED!\""
  String Constant2 : StringConstant  String="\"Horn And Lights are ON!\""
  Switch : Switch  Criteria=u2 ~= 0
  Switch1 : Switch  Criteria=u2 ~= 0
  Toggle Switch : ToggleSwitchBlock
      settings: Values={{'Off', 'On'}, [0 1]}
  tag scope: Alarm_ARMED=global, Disarmed=global, Prealarm_ARMED=global
  wires:
  [Ignition] -> Compare To Constant2/1, AND/1
  AND/1 -> Compare To Constant/1
  [CAR_ON] -> AND/2
  ARMED/1(data1) -> AND1/3, Compare To Constant3/1
  data2/1 -> Compare To Zero1/1, AND/3
  Compare To Constant2/1 -> AND1/1
  [RKE] -> AND1/2, Compare To Zero/1, AND2/2  "RKE"
  AND1/1 -> Switch/2
  String Constant/1 -> Switch/1
  Switch/1 -> [Disarmed]
  Pre_Alarm/1(data1) -> Switch1/2
  String Constant2/1 -> Switch1/1
  Compare To Constant/1 -> AND2/1
  Compare To Constant3/1 -> [Alarm_ARMED]
  AND2/1 -> ARMED/1(data)
  Compare To Zero/1 -> AND3/1
  AND3/1 -> Pre_Alarm/1(data)
  Compare To Zero1/1 -> AND3/2
  Switch1/1 -> [Prealarm_ARMED]

== system Automated_features/MODULES/WIPER_CONTROL/Atomic Subsystem ==
  Inport : Inport
  Clock : Clock
      settings: Decimation=5
  Compare To Constant : simulink/Logic and Bit Operations/Compare To Constant  relop===  const=1  OutDataTypeStr=boolean
  Compare To Constant5 : simulink/Logic and Bit Operations/Compare To Constant  relop===  const=1  OutDataTypeStr=boolean
  Gain : Gain  Gain=10
  Relational Operator : RelationalOperator  Operator=<  OutDataTypeStr=boolean  RndMeth=Simplest
  tag scope: BW_Display=global
  wires:
  Compare To Constant5/1 -> [BW_Display]
  Inport/1 -> Compare To Constant/1
  Gain/1 -> Relational Operator/2
  Clock/1 -> Relational Operator/1
  Relational Operator/1 -> Compare To Constant5/1
  Compare To Constant/1 -> Gain/1

== system Automated_features/MODULES/WIPER_CONTROL/Atomic Subsystem1 ==
  Inport : Inport
  Auto_Modes : Subsystem
  Display : Display
  Manual_mode : Subsystem
  wires:
  [FW_Modes] -> Manual_mode/1(In1), Auto_Modes/1(In1)
  Inport/1 -> Display/1

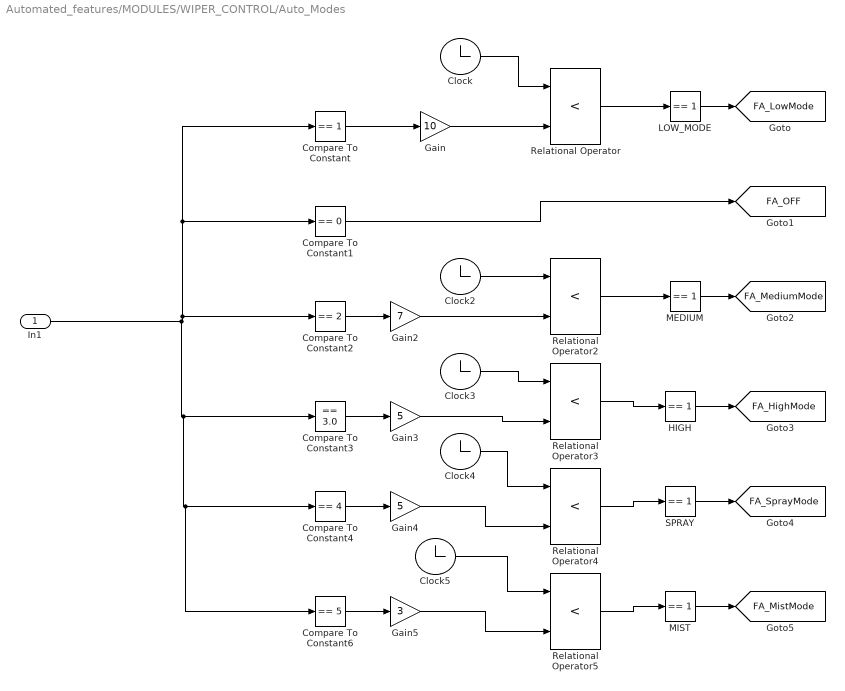
== system Automated_features/MODULES/WIPER_CONTROL/Auto_Modes ==
  In1 : Inport
  Clock{,2..5} (5 alike) : Clock
      settings: Decimation=5
  Compare To Constant : simulink/Logic and Bit Operations/Compare To Constant  relop===  const=1  OutDataTypeStr=boolean
  Compare To Constant1 : simulink/Logic and Bit Operations/Compare To Constant  relop===  const=0  OutDataTypeStr=boolean
  Compare To Constant2 : simulink/Logic and Bit Operations/Compare To Constant  relop===  const=2  OutDataTypeStr=boolean
  Compare To Constant3 : simulink/Logic and Bit Operations/Compare To Constant  relop===  const=3.0  OutDataTypeStr=boolean
  Compare To Constant4 : simulink/Logic and Bit Operations/Compare To Constant  relop===  const=4  OutDataTypeStr=boolean
  Compare To Constant6 : simulink/Logic and Bit Operations/Compare To Constant  relop===  const=5  OutDataTypeStr=boolean
  Gain : Gain  Gain=10
  Gain2 : Gain  Gain=7
  Gain3 : Gain  Gain=5
  Gain4 : Gain  Gain=5
  Gain5 : Gain  Gain=3
  HIGH : simulink/Logic and Bit Operations/Compare To Constant  relop===  const=1  OutDataTypeStr=boolean
  LOW_MODE : simulink/Logic and Bit Operations/Compare To Constant  relop===  const=1  OutDataTypeStr=boolean
  MEDIUM : simulink/Logic and Bit Operations/Compare To Constant  relop===  const=1  OutDataTypeStr=boolean
  MIST : simulink/Logic and Bit Operations/Compare To Constant  relop===  const=1  OutDataTypeStr=boolean
  Relational Operator{,2..5} (5 alike) : RelationalOperator  Operator=<  OutDataTypeStr=boolean  RndMeth=Simplest
  SPRAY : simulink/Logic and Bit Operations/Compare To Constant  relop===  const=1  OutDataTypeStr=boolean
  tag scope: FA_HighMode=global, FA_LowMode=global, FA_MediumMode=global, FA_MistMode=global, FA_OFF=global, FA_SprayMode=global
  wires:
  In1/1 -> Compare To Constant6/1, Compare To Constant4/1, Compare To Constant3/1, Compare To Constant2/1, Compare To Constant/1, Compare To Constant1/1
  Clock/1 -> Relational Operator/1
  Relational Operator/1 -> LOW_MODE/1
  Gain/1 -> Relational Operator/2
  Compare To Constant/1 -> Gain/1
  Clock2/1 -> Relational Operator2/1
  Gain2/1 -> Relational Operator2/2
  Compare To Constant2/1 -> Gain2/1
  Clock3/1 -> Relational Operator3/1
  Gain3/1 -> Relational Operator3/2
  Compare To Constant3/1 -> Gain3/1
  Gain4/1 -> Relational Operator4/2
  Clock4/1 -> Relational Operator4/1
  Compare To Constant4/1 -> Gain4/1
  LOW_MODE/1 -> [FA_LowMode]
  MEDIUM/1 -> [FA_MediumMode]
  Relational Operator2/1 -> MEDIUM/1
  HIGH/1 -> [FA_HighMode]
  Relational Operator3/1 -> HIGH/1
  SPRAY/1 -> [FA_SprayMode]
  Relational Operator4/1 -> SPRAY/1
  Compare To Constant1/1 -> [FA_OFF]
  Relational Operator5/1 -> MIST/1
  Gain5/1 -> Relational Operator5/2
  Clock5/1 -> Relational Operator5/1
  MIST/1 -> [FA_MistMode]
  Compare To Constant6/1 -> Gain5/1

== system Automated_features/MODULES/WIPER_CONTROL/Back_Windshield ==
  Lamp : LampBlock

== system Automated_features/MODULES/WIPER_CONTROL/Front_Windshield ==
  Enable : EnablePort
  Auto_Modes : Subsystem
  Manual_mode : Subsystem
  Rotary Switch : RotarySwitchBlock  Commented=on
      settings: Values={{'Off', 'Low', 'Medium', 'High', 'Spray', 'Manual', 'MistMode'}, [0 1 2 3 4 5 6]}
  wires:
  [FW_Modes] -> Manual_mode/1(In1), Auto_Modes/1(In1)

== system Automated_features/MODULES/WIPER_CONTROL/Manual_mode ==
  In1 : Inport
  Bw30_60 : Logic  IconShape=distinctive  AllPortsSameDT=off  OutDataTypeStr=boolean
  Bw60_100 : Logic  IconShape=distinctive  AllPortsSameDT=off  OutDataTypeStr=boolean
  Compare To Constant1 : simulink/Logic and Bit Operations/Compare To Constant  relop=>  const=30  OutDataTypeStr=boolean
  Compare To Constant2 : simulink/Logic and Bit Operations/Compare To Constant  relop=<=  const=60  OutDataTypeStr=boolean
  Compare To Constant3 : simulink/Logic and Bit Operations/Compare To Constant  relop=>  const=60  OutDataTypeStr=boolean
  Compare To Constant4 : simulink/Logic and Bit Operations/Compare To Constant  relop=<=  const=100  OutDataTypeStr=boolean
  Display : Display
  LessThan30 : simulink/Logic and Bit Operations/Compare To Constant  relop=<=  const=30  OutDataTypeStr=boolean
  Slider : SliderBlock
  String Constant : StringConstant  String="\"Undefined!\""
  Switch : Switch  Criteria=u2 > Threshold  Threshold=5
  tag scope: FM_Bw30_60=global, FM_Bw60_100=global, FM_lessthan30=global
  wires:
  Compare To Constant1/1 -> Bw30_60/1
  Bw30_60/1 -> [FM_Bw30_60]
  [FC_ManualInput] -> Compare To Constant4/1, Compare To Constant3/1, Compare To Constant2/1, Compare To Constant1/1, LessThan30/1, Switch/1
  Compare To Constant4/1 -> Bw60_100/2
  LessThan30/1 -> [FM_lessthan30]
  Switch/1 -> Display/1
  Compare To Constant3/1 -> Bw60_100/1
  Bw60_100/1 -> [FM_Bw60_100]
  Compare To Constant2/1 -> Bw30_60/2
  In1/1 -> Switch/2
  String Constant/1 -> Switch/3

== system Automated_features/MODULES/WIPER_CONTROL/Wiper_Control ==
  Inport : Inport
  AND : Logic  IconShape=distinctive  AllPortsSameDT=off  OutDataTypeStr=boolean
  AND1 : Logic  IconShape=distinctive  AllPortsSameDT=off  OutDataTypeStr=boolean
  Atomic Subsystem : Subsystem  TreatAsAtomicUnit=on
  Atomic Subsystem1 : Subsystem  TreatAsAtomicUnit=on
  Back switch : SliderSwitchBlock  Commented=on
      settings: Values={{'Off', 'On'}, [0 1]}
  Back_Windshield : Subsystem  Commented=on  TreatAsAtomicUnit=on
  Front switch : SliderSwitchBlock  Commented=on
      settings: Values={{'Off', 'On'}, [0 1]}
  Front_Windshield : Subsystem  Commented=on  TreatAsAtomicUnit=on
  wires:
  Inport/1 -> AND1/2, AND/2
  [WC_FrontS] -> AND/1
  [WC_BackS] -> AND1/1
  AND1/1 -> Atomic Subsystem/1(Inport)
  AND/1 -> Atomic Subsystem1/1(Inport)

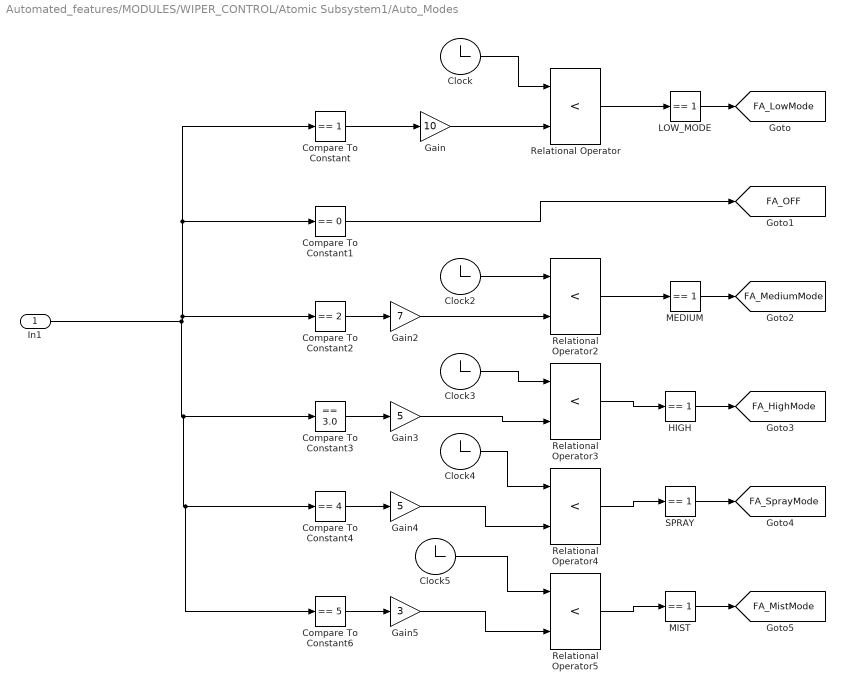
== system Automated_features/MODULES/WIPER_CONTROL/Atomic Subsystem1/Auto_Modes ==
  In1 : Inport
  Clock{,2..5} (5 alike) : Clock
      settings: Decimation=5
  Compare To Constant : simulink/Logic and Bit Operations/Compare To Constant  relop===  const=1  OutDataTypeStr=boolean
  Compare To Constant1 : simulink/Logic and Bit Operations/Compare To Constant  relop===  const=0  OutDataTypeStr=boolean
  Compare To Constant2 : simulink/Logic and Bit Operations/Compare To Constant  relop===  const=2  OutDataTypeStr=boolean
  Compare To Constant3 : simulink/Logic and Bit Operations/Compare To Constant  relop===  const=3.0  OutDataTypeStr=boolean
  Compare To Constant4 : simulink/Logic and Bit Operations/Compare To Constant  relop===  const=4  OutDataTypeStr=boolean
  Compare To Constant6 : simulink/Logic and Bit Operations/Compare To Constant  relop===  const=5  OutDataTypeStr=boolean
  Gain : Gain  Gain=10
  Gain2 : Gain  Gain=7
  Gain3 : Gain  Gain=5
  Gain4 : Gain  Gain=5
  Gain5 : Gain  Gain=3
  HIGH : simulink/Logic and Bit Operations/Compare To Constant  relop===  const=1  OutDataTypeStr=boolean
  LOW_MODE : simulink/Logic and Bit Operations/Compare To Constant  relop===  const=1  OutDataTypeStr=boolean
  MEDIUM : simulink/Logic and Bit Operations/Compare To Constant  relop===  const=1  OutDataTypeStr=boolean
  MIST : simulink/Logic and Bit Operations/Compare To Constant  relop===  const=1  OutDataTypeStr=boolean
  Relational Operator{,2..5} (5 alike) : RelationalOperator  Operator=<  OutDataTypeStr=boolean  RndMeth=Simplest
  SPRAY : simulink/Logic and Bit Operations/Compare To Constant  relop===  const=1  OutDataTypeStr=boolean
  tag scope: FA_HighMode=global, FA_LowMode=global, FA_MediumMode=global, FA_MistMode=global, FA_OFF=global, FA_SprayMode=global
  wires:
  In1/1 -> Compare To Constant6/1, Compare To Constant4/1, Compare To Constant3/1, Compare To Constant2/1, Compare To Constant/1, Compare To Constant1/1
  Clock/1 -> Relational Operator/1
  Relational Operator/1 -> LOW_MODE/1
  Gain/1 -> Relational Operator/2
  Compare To Constant/1 -> Gain/1
  Clock2/1 -> Relational Operator2/1
  Gain2/1 -> Relational Operator2/2
  Compare To Constant2/1 -> Gain2/1
  Clock3/1 -> Relational Operator3/1
  Gain3/1 -> Relational Operator3/2
  Compare To Constant3/1 -> Gain3/1
  Gain4/1 -> Relational Operator4/2
  Clock4/1 -> Relational Operator4/1
  Compare To Constant4/1 -> Gain4/1
  LOW_MODE/1 -> [FA_LowMode]
  MEDIUM/1 -> [FA_MediumMode]
  Relational Operator2/1 -> MEDIUM/1
  HIGH/1 -> [FA_HighMode]
  Relational Operator3/1 -> HIGH/1
  SPRAY/1 -> [FA_SprayMode]
  Relational Operator4/1 -> SPRAY/1
  Compare To Constant1/1 -> [FA_OFF]
  Relational Operator5/1 -> MIST/1
  Gain5/1 -> Relational Operator5/2
  Clock5/1 -> Relational Operator5/1
  MIST/1 -> [FA_MistMode]
  Compare To Constant6/1 -> Gain5/1

== system Automated_features/MODULES/WIPER_CONTROL/Atomic Subsystem1/Manual_mode ==
  In1 : Inport
  Bw30_60 : Logic  IconShape=distinctive  AllPortsSameDT=off  OutDataTypeStr=boolean
  Bw60_100 : Logic  IconShape=distinctive  AllPortsSameDT=off  OutDataTypeStr=boolean
  Compare To Constant1 : simulink/Logic and Bit Operations/Compare To Constant  relop=>  const=30  OutDataTypeStr=boolean
  Compare To Constant2 : simulink/Logic and Bit Operations/Compare To Constant  relop=<=  const=60  OutDataTypeStr=boolean
  Compare To Constant3 : simulink/Logic and Bit Operations/Compare To Constant  relop=>  const=60  OutDataTypeStr=boolean
  Compare To Constant4 : simulink/Logic and Bit Operations/Compare To Constant  relop=<=  const=100  OutDataTypeStr=boolean
  Display : Display
  LessThan30 : simulink/Logic and Bit Operations/Compare To Constant  relop=<=  const=30  OutDataTypeStr=boolean
  Slider : SliderBlock
  String Constant : StringConstant  String="\"Undefined!\""
  Switch : Switch  Criteria=u2 > Threshold  Threshold=5
  tag scope: FM_Bw30_60=global, FM_Bw60_100=global, FM_lessthan30=global
  wires:
  Compare To Constant1/1 -> Bw30_60/1
  Bw30_60/1 -> [FM_Bw30_60]
  [FC_ManualInput] -> Compare To Constant4/1, Compare To Constant3/1, Compare To Constant2/1, Compare To Constant1/1, LessThan30/1, Switch/1
  Compare To Constant4/1 -> Bw60_100/2
  LessThan30/1 -> [FM_lessthan30]
  Switch/1 -> Display/1
  Compare To Constant3/1 -> Bw60_100/1
  Bw60_100/1 -> [FM_Bw60_100]
  Compare To Constant2/1 -> Bw30_60/2
  In1/1 -> Switch/2
  String Constant/1 -> Switch/3

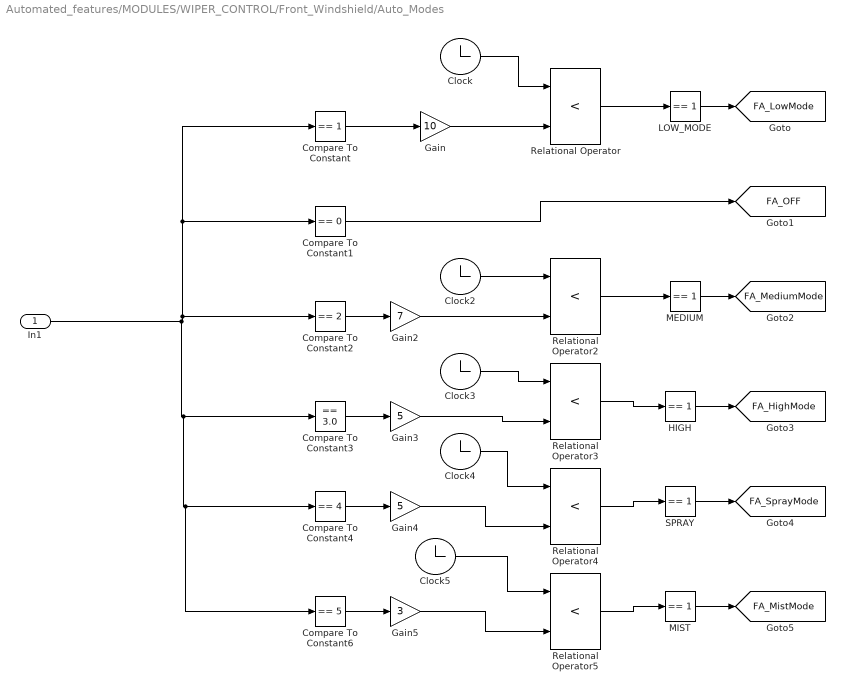
== system Automated_features/MODULES/WIPER_CONTROL/Front_Windshield/Auto_Modes ==
  In1 : Inport
  Clock{,2..5} (5 alike) : Clock
      settings: Decimation=5
  Compare To Constant : simulink/Logic and Bit Operations/Compare To Constant  relop===  const=1  OutDataTypeStr=boolean
  Compare To Constant1 : simulink/Logic and Bit Operations/Compare To Constant  relop===  const=0  OutDataTypeStr=boolean
  Compare To Constant2 : simulink/Logic and Bit Operations/Compare To Constant  relop===  const=2  OutDataTypeStr=boolean
  Compare To Constant3 : simulink/Logic and Bit Operations/Compare To Constant  relop===  const=3.0  OutDataTypeStr=boolean
  Compare To Constant4 : simulink/Logic and Bit Operations/Compare To Constant  relop===  const=4  OutDataTypeStr=boolean
  Compare To Constant6 : simulink/Logic and Bit Operations/Compare To Constant  relop===  const=5  OutDataTypeStr=boolean
  Gain : Gain  Gain=10
  Gain2 : Gain  Gain=7
  Gain3 : Gain  Gain=5
  Gain4 : Gain  Gain=5
  Gain5 : Gain  Gain=3
  HIGH : simulink/Logic and Bit Operations/Compare To Constant  relop===  const=1  OutDataTypeStr=boolean
  LOW_MODE : simulink/Logic and Bit Operations/Compare To Constant  relop===  const=1  OutDataTypeStr=boolean
  MEDIUM : simulink/Logic and Bit Operations/Compare To Constant  relop===  const=1  OutDataTypeStr=boolean
  MIST : simulink/Logic and Bit Operations/Compare To Constant  relop===  const=1  OutDataTypeStr=boolean
  Relational Operator{,2..5} (5 alike) : RelationalOperator  Operator=<  OutDataTypeStr=boolean  RndMeth=Simplest
  SPRAY : simulink/Logic and Bit Operations/Compare To Constant  relop===  const=1  OutDataTypeStr=boolean
  tag scope: FA_HighMode=global, FA_LowMode=global, FA_MediumMode=global, FA_MistMode=global, FA_OFF=global, FA_SprayMode=global
  wires:
  In1/1 -> Compare To Constant6/1, Compare To Constant4/1, Compare To Constant3/1, Compare To Constant2/1, Compare To Constant/1, Compare To Constant1/1
  Clock/1 -> Relational Operator/1
  Relational Operator/1 -> LOW_MODE/1
  Gain/1 -> Relational Operator/2
  Compare To Constant/1 -> Gain/1
  Clock2/1 -> Relational Operator2/1
  Gain2/1 -> Relational Operator2/2
  Compare To Constant2/1 -> Gain2/1
  Clock3/1 -> Relational Operator3/1
  Gain3/1 -> Relational Operator3/2
  Compare To Constant3/1 -> Gain3/1
  Gain4/1 -> Relational Operator4/2
  Clock4/1 -> Relational Operator4/1
  Compare To Constant4/1 -> Gain4/1
  LOW_MODE/1 -> [FA_LowMode]
  MEDIUM/1 -> [FA_MediumMode]
  Relational Operator2/1 -> MEDIUM/1
  HIGH/1 -> [FA_HighMode]
  Relational Operator3/1 -> HIGH/1
  SPRAY/1 -> [FA_SprayMode]
  Relational Operator4/1 -> SPRAY/1
  Compare To Constant1/1 -> [FA_OFF]
  Relational Operator5/1 -> MIST/1
  Gain5/1 -> Relational Operator5/2
  Clock5/1 -> Relational Operator5/1
  MIST/1 -> [FA_MistMode]
  Compare To Constant6/1 -> Gain5/1

== system Automated_features/MODULES/WIPER_CONTROL/Front_Windshield/Manual_mode ==
  In1 : Inport
  Bw30_60 : Logic  IconShape=distinctive  AllPortsSameDT=off  OutDataTypeStr=boolean
  Bw60_100 : Logic  IconShape=distinctive  AllPortsSameDT=off  OutDataTypeStr=boolean
  Compare To Constant1 : simulink/Logic and Bit Operations/Compare To Constant  relop=>  const=30  OutDataTypeStr=boolean
  Compare To Constant2 : simulink/Logic and Bit Operations/Compare To Constant  relop=<=  const=60  OutDataTypeStr=boolean
  Compare To Constant3 : simulink/Logic and Bit Operations/Compare To Constant  relop=>  const=60  OutDataTypeStr=boolean
  Compare To Constant4 : simulink/Logic and Bit Operations/Compare To Constant  relop=<=  const=100  OutDataTypeStr=boolean
  Display : Display
  LessThan30 : simulink/Logic and Bit Operations/Compare To Constant  relop=<=  const=30  OutDataTypeStr=boolean
  Slider : SliderBlock
  String Constant : StringConstant  String="\"Undefined!\""
  Switch : Switch  Criteria=u2 > Threshold  Threshold=5
  tag scope: FM_Bw30_60=global, FM_Bw60_100=global, FM_lessthan30=global
  wires:
  Compare To Constant1/1 -> Bw30_60/1
  Bw30_60/1 -> [FM_Bw30_60]
  [FC_ManualInput] -> Compare To Constant4/1, Compare To Constant3/1, Compare To Constant2/1, Compare To Constant1/1, LessThan30/1, Switch/1
  Compare To Constant4/1 -> Bw60_100/2
  LessThan30/1 -> [FM_lessthan30]
  Switch/1 -> Display/1
  Compare To Constant3/1 -> Bw60_100/1
  Bw60_100/1 -> [FM_Bw60_100]
  Compare To Constant2/1 -> Bw30_60/2
  In1/1 -> Switch/2
  String Constant/1 -> Switch/3

== system Automated_features/MODULES/WIPER_CONTROL/Wiper_Control/Atomic Subsystem ==
  Inport : Inport
  Clock : Clock
      settings: Decimation=5
  Compare To Constant : simulink/Logic and Bit Operations/Compare To Constant  relop===  const=1  OutDataTypeStr=boolean
  Compare To Constant5 : simulink/Logic and Bit Operations/Compare To Constant  relop===  const=1  OutDataTypeStr=boolean
  Gain : Gain  Gain=10
  Relational Operator : RelationalOperator  Operator=<  OutDataTypeStr=boolean  RndMeth=Simplest
  tag scope: BW_Display=global
  wires:
  Compare To Constant5/1 -> [BW_Display]
  Inport/1 -> Compare To Constant/1
  Gain/1 -> Relational Operator/2
  Clock/1 -> Relational Operator/1
  Relational Operator/1 -> Compare To Constant5/1
  Compare To Constant/1 -> Gain/1

== system Automated_features/MODULES/WIPER_CONTROL/Wiper_Control/Atomic Subsystem1 ==
  Inport : Inport
  Auto_Modes : Subsystem
  Display : Display
  Manual_mode : Subsystem
  wires:
  [FW_Modes] -> Manual_mode/1(In1), Auto_Modes/1(In1)
  Inport/1 -> Display/1

== system Automated_features/MODULES/WIPER_CONTROL/Wiper_Control/Back_Windshield ==
  Lamp : LampBlock

== system Automated_features/MODULES/WIPER_CONTROL/Wiper_Control/Front_Windshield ==
  Enable : EnablePort
  Auto_Modes : Subsystem
  Manual_mode : Subsystem
  Rotary Switch : RotarySwitchBlock  Commented=on
      settings: Values={{'Off', 'Low', 'Medium', 'High', 'Spray', 'Manual', 'MistMode'}, [0 1 2 3 4 5 6]}
  wires:
  [FW_Modes] -> Manual_mode/1(In1), Auto_Modes/1(In1)
